simulink subsystem "startQuaternionFlipper"  (R2021a)
settings: Solver=VariableStepAuto  StartTime=0.0  StopTime=10.0  RelTol=1e-3
settings Model: Creator=noraw  LastModifiedBy=noraw

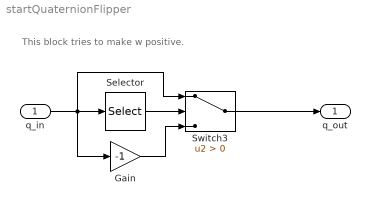
== system startQuaternionFlipper ==
  note: This block tries to make w positive.
  q_in : Inport
  Gain : Gain  Gain=-1
  Selector : Selector  InputPortWidth=4  IndexOptions=Index vector (dialog)  Indices=[1]  OutputSizes=1
  Switch3 : Switch  Criteria=u2 > Threshold  ZeroCross=off
  q_out : Outport
  wires:
  Gain/1 -> Switch3/3
  Selector/1 -> Switch3/2
  q_in/1 -> Switch3/1, Selector/1, Gain/1
  Switch3/1 -> q_out/1
